simulink model "entire_model"  (R2023b)
settings: Solver=VariableStepAuto  StartTime=0.0  StopTime=600  RelTol=1e-3
values from neighbouring files (symbols this model uses):
  Gamma = diag([ 10*ga, 10*ga, 10*ga, 10*ga, 10*ga])    [CA1_params.m]
  theta_bar_star = [K_star, -G1(3), -G1(2), -Fbar(4), -Fbar(3)]    [CA1_params.m]
  Tp = [1 2*zeta*wn wn^2]    [CA1_params.m]
settings Model: Creator=john  LastModifiedBy=john

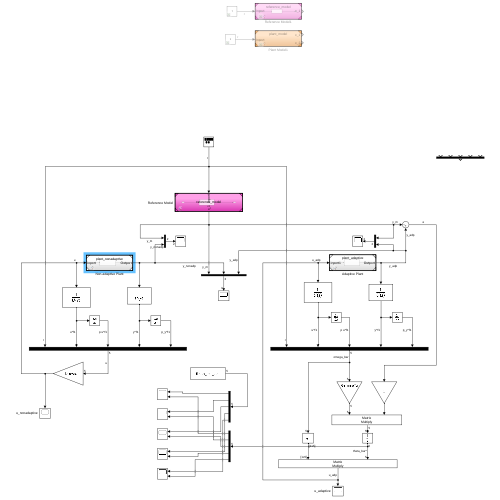
[thumbnail: Simulink's stored preview of the top-level diagram]
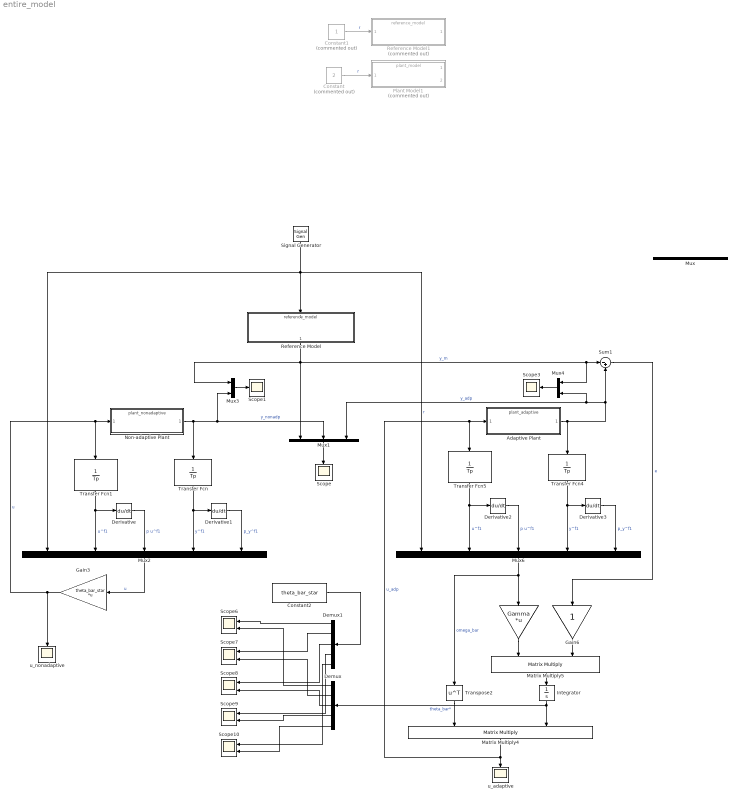
== system entire_model ==
  " " : Gain  Gain=Gamma  Multiplication=Matrix(K*u)
  Adaptive Plant : ModelReference  ModelNameDialog=plant_adaptive.slx  SimulationMode=Normal  ModelReferenceVersion=1.11
  Constant : Constant  Commented=on  Value=2
  Constant1 : Constant  Commented=on
  Constant2 : Constant  Value=theta_bar_star
  Demux : Demux  Outputs=5
  Demux1 : Demux  Outputs=5
  Derivative{,1..3} (4 alike) : Derivative
  Gain3 : Gain  Gain=theta_bar_star  Multiplication=Matrix(K*u) (u vector)
  Gain6 : Gain
  Integrator : Integrator
  Matrix Multiply4 : Product  Multiplication=Matrix(*)
  Matrix Multiply5 : Product  Multiplication=Matrix(*)
  Mux : Mux  Inputs=5
  Mux1 : Mux  Inputs=3
  Mux2 : Mux  Inputs=5
  Mux3 : Mux  Inputs=2
  Mux4 : Mux  Inputs=2
  Mux6 : Mux  Inputs=5
  Non-adaptive Plant : ModelReference  ModelNameDialog=plant_nonadaptive.slx  SimulationMode=Normal  ModelReferenceVersion=1.4
  Plant Model1 : ModelReference  Commented=on  ModelNameDialog=plant_model.slx  SimulationMode=Normal  ModelReferenceVersion=1.14
  Reference Model : ModelReference  ModelNameDialog=reference_model.slx  SimulationMode=Normal  ModelReferenceVersion=1.13
  Reference Model1 : ModelReference  Commented=on  ModelNameDialog=reference_model.slx  SimulationMode=Normal  ModelReferenceVersion=1.13
  Scope : Scope
  Scope1 : Scope
  Scope{6..10} (5 alike) : Scope  NumInputPorts=2
  Scope3 : Scope
  Signal Generator : SignalGenerator  WaveForm=square  Frequency=0.1  Units=rad/sec
  Sum1 : Sum  Inputs=|-+
  Transfer Fcn{,1,4..5} (4 alike) : TransferFcn  Numerator=1  Denominator=Tp
  Transpose2 : Math  Operator=transpose
  u_adaptive : Scope
  u_nonadaptive : Scope
  wires:
  Signal Generator/1 -> Mux2/1, Mux6/1, Reference Model/1  "r"
  Constant1/1 -> Reference Model1/1  "r"
  Constant/1 -> Plant Model1/1  "r"
  Non-adaptive Plant/1 -> Mux1/2, Mux3/2, Transfer Fcn/1  "y_nonadp"
  Gain3/1 -> Transfer Fcn1/1, Non-adaptive Plant/1, u_nonadaptive/1  "u"
  Transfer Fcn/1 -> Derivative1/1, Mux2/4  "y^f1"
  Mux1/1 -> Scope/1
  Mux3/1 -> Scope1/1
  Reference Model/1 -> Mux1/1, Mux3/1, Mux4/1, Sum1/1  "y_m"
  Mux4/1 -> Scope3/1
  Integrator/1 -> Matrix Multiply4/2, Demux/1  "theta_bar*"
  Matrix Multiply5/1 -> Integrator/1
  " "/1 -> Matrix Multiply5/1
  Gain6/1 -> Matrix Multiply5/2
  Mux6/1 -> Transpose2/1, " "/1  "omega_bar"
  Transfer Fcn1/1 -> Derivative/1, Mux2/2  "u^f1"
  Derivative/1 -> Mux2/3  "p u^f1"
  Derivative1/1 -> Mux2/5  "p_y^f1"
  Mux2/1 -> Gain3/1  "u"
  Transfer Fcn5/1 -> Derivative2/1, Mux6/2  "u^f1"
  Adaptive Plant/1 -> Mux4/2, Mux1/3, Sum1/2, Transfer Fcn4/1  "y_adp"
  Derivative3/1 -> Mux6/5  "p_y^f1"
  Derivative2/1 -> Mux6/3  "p u^f1"
  Transfer Fcn4/1 -> Derivative3/1, Mux6/4  "y^f1"
  Matrix Multiply4/1 -> u_adaptive/1, Adaptive Plant/1, Transfer Fcn5/1  "u_adp"
  Sum1/1 -> Gain6/1  "e"
  Transpose2/1 -> Matrix Multiply4/1
  Constant2/1 -> Demux1/1
  Demux1/1 -> Scope6/1
  Demux/1 -> Scope6/2
  Demux1/2 -> Scope7/1
  Demux/2 -> Scope7/2
  Demux1/3 -> Scope8/1
  Demux/3 -> Scope8/2
  Demux1/4 -> Scope9/1
  Demux/4 -> Scope9/2
  Demux1/5 -> Scope10/1
  Demux/5 -> Scope10/2
